simulink model "hexa_CAD_FxQDiff_ASGSM"  (R2024a)
settings: Solver=ode4  StartTime=0.0  StopTime=60  FixedStep=0.01  RelTol=1e-3
undefined symbols (not defined in the file or in its folder): F, Light, MIL, smiData, X, Y, Z
libraries: sm_lib x166, nesl_utility x29, dspobslib x16, sharedtransform x6, aerolibutil x6, simulink x4, sharedutil x2, matrix_library x1, robotcorelib x1, aerolibwind2 x1
(part 2 of 5)

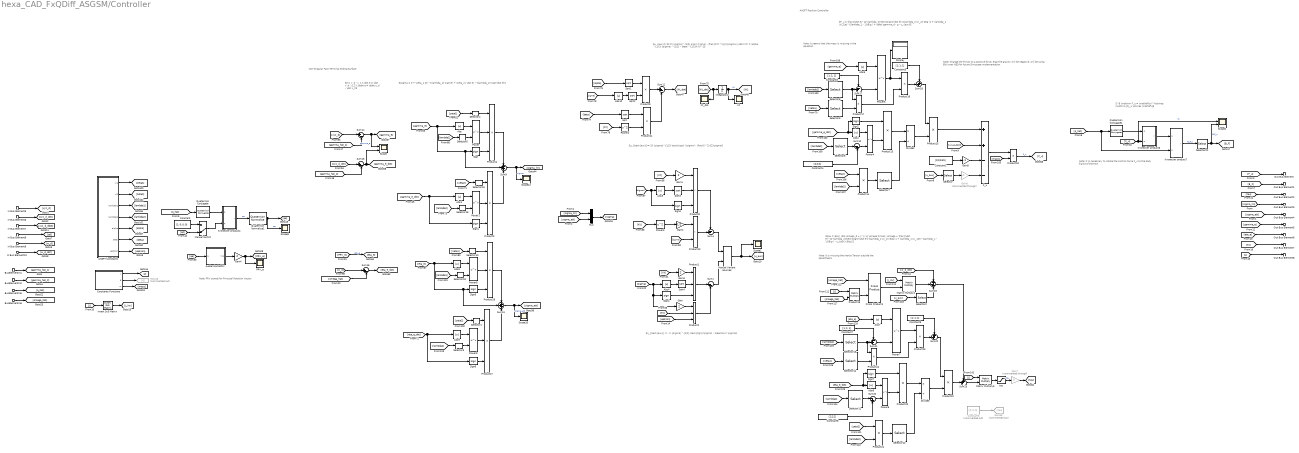
== system hexa_CAD_FxQDiff_ASGSM/Controller ==
  note: $u_{\text{aux}}=-2K |\sigma|^{1/2} \text{sign} (\sigma) - \frac{K^2}{2}\sigma$
  note: $u_{\text{aux}} = - K |\sigma| ^{1/2} \text{sign}(\sigma) - 2\epsilon K \sigma$
  note: Note: PRV stands for Principal Rotation
      | Vector.
  note: $e = x_d - x_1 \\ \dot e = \dot x_d - x_2 \\ \ddot e = \ddot x_d - \dot x_2$
  note: Non-Singular Fast Terminal Sliding Surface
  note: $\sigma = e + \zeta_1 |e| ^{\lambda_1} sign(e) + \zeta_2 | \dot e| ^{\lambda_2} sign(\dot e)$
  note: $F_u = \frac{|\dot e|^{2-\lambda_2}\text{sign}(\dot e)}{\lambda_2 \xi_2} \Big (1 + \lambda_1 \xi_1|e|^{\lambda_1 - 1}\Big ) + \ddot \gamma_d - g - u_{aux}$
  note: Note: It seems that the mass is missing in
      | the equation.
  note: $\tau = \Big [ \dot \omega_d + J^{-1} \omega \times J \omega + \frac{|\dot e|^{2-\lambda_2}\text{sign}(\dot e)}{\lambda_2 \xi_2} \Big (1 + \lambda_1 \xi_1|e|^{\lambda_1 - 1}\Big ) - u_{aux} \Big ]$
  note: Note: Change the Thrust to a positive force, ergo the gravity will be negative,
      | will be using ENU over NED for future Simscape implementation.
  note: $^B \mathrm F_u = \mathbf{q}^*\otimes \mathrm{F}_u \otimes \mathbf q$
  note: ANSFT Position Controller
  note: Note: It is missing the Inertia Tensor outside
      | the parenthesis
  note: Note: It is necessary to rotate the control Force F_u
      | to the body frame of the FAH.
  note: $u_{aux}=-2K(t) |\sigma|^{1/2} sign (\sigma) - \frac{K(t)^2}{2}\sigma \\ \dot K(t) = \alpha ^{1/2} |\sigma| ^{1/2} - \beta ^{1/2}K(t)^2$
  In Bus Element5 : Inport  PortName=chi_d  Element=xyz_d
  In Bus Element6 : Inport  PortName=chi_d  Element=xyz_d_dot
  In Bus Element7 : Inport  PortName=chi_d  Element=xyz_d_ddot
  In Bus Element8 : Inport  PortName=chi_d  Element=qd
  In Bus Element9 : Inport  PortName=chi_d  Element=w_d
  In Bus Element10 : Inport  PortName=chi_d  Element=w_d_dot
  BusElementIn1 : Inport  Port=2  PortName=q_hat  Element=gamma_hat
  BusElementIn2 : Inport  Port=2  PortName=q_hat  Element=gamma_dot_hat
  BusElementIn5 : Inport  Port=2  PortName=q_hat  Element=q_hat
  BusElementIn6 : Inport  Port=2  PortName=q_hat  Element=omega_hat
  ANSFT Constants : MATLAB Function  TreatAsAtomicUnit=on
  Abs{,1..10} (11 alike) : Abs  SaturateOnIntegerOverflow=off
  Constant : Constant  Value=[1; 0; 0; 0]
  Constant1 : Constant  Value=[0;0;9.81]
  Constant{3,5,7,9} (4 alike) : Constant  Value=[1; 1; 1]
  Constant4 : Constant  Value=[2;2;2]
  Constant6 : Constant  Commented=on  Value=[0; 0; 0]
  Constant8 : Constant  Value=[2;2;2]
  Constants Functions : MATLAB Function  TreatAsAtomicUnit=on
  Cross Product1 : matrix_library/Cross Product
  Display : Display
  Divide2 : Product  Inputs=*/
  Divide3 : Product  Inputs=*/
  F_u : Sum  Inputs=++--
  Gain{,1,3..4} (4 alike) : Gain  Gain=2
  Gain2 : Gain  Gain=1/2
  Gain5 : Gain  Gain=-1
  Gain6 : Gain  Commented=through  Gain=-1
  Gain7 : Gain  Commented=through  Gain=0
  Goto18 : Goto  Commented=on  GotoTag=g
  Goto59 : Goto  Commented=on  GotoTag=tau
  Integrator4 : Integrator  InitialCondition=[0;0;0; 0; 0; 0]
  Invert 3x3 Matrix : aerolibutil/Invert  3x3 Matrix
  Kronecker product4 : Subsystem
  Kronecker product6 : Subsystem
  Kronecker product7 : Subsystem
  Kt : Scope
  Kt_dot : Scope
  Manual Variant Source3 : simulink/Signal Routing/Manual Variant Source  NumChoices=2  LabelModeActiveChoice=V_2
  Manual Switch : ManualSwitch  CurrentSetting=0
  Matrix Multiply2 : Product  Multiplication=Matrix(*)
  Matrix Multiply5 : Product  Multiplication=Matrix(*)
  Mux : Mux  Inputs=2
  PRV_e : Scope
  Power{,1,4..9} (8 alike) : Math  Operator=pow
  Power2 : Math  Operator=square
  Power3 : Math  Operator=square
  Product{1..4,8,26..27} (7 alike) : Product  Inputs=3
  Product{9..11,13..18,20..24} (14 alike) : Product
  Product19 : Product  Multiplication=Matrix(*)
  Quaternion Conjugate : aerolibutil/Quaternion Conjugate
  Quaternion Conjugate1 : aerolibutil/Quaternion Conjugate
  Quaternion Normalize1 : sharedutil/Quaternion Normalize  aMode=aMode
  Scope : Scope  NumInputPorts=2
  Scope{1,8,10,12} (4 alike) : Scope
  Scope2 : Scope  NumInputPorts=2
  Selector{,4..9,15..16} (9 alike) : Selector  InputPortWidth=6  IndexOptions=Index vector (dialog)  Indices=[1:3]  OutputSizes=1
  Selector{1..3,10..14,18} (9 alike) : Selector  InputPortWidth=6  IndexOptions=Index vector (dialog)  Indices=[4:6]  OutputSizes=1
  Selector22 : Selector  InputPortWidth=4  IndexOptions=Index vector (dialog)  Indices=[2:4]  OutputSizes=1
  Sign{,1..7} (8 alike) : Signum
  Sqrt{,1..4} (5 alike) : Sqrt
  Sum1 : Sum  Inputs=|--
  Sum10 : Sum  Inputs=|-+
  Sum{11,14..16} (4 alike) : Sum  Inputs=|+-
  Sum17 : Sum  Inputs=-+|
  Sum18 : Sum  Inputs=++|
  Sum19 : Sum  Inputs=+--
  Sum20 : Sum  Inputs=|-+
  Sum21 : Sum  Inputs=-+|
  Sum22 : Sum  Inputs=++|
  Sum23 : Sum  Inputs=++|
  Sum24 : Sum  Inputs=+++
  Sum4 : Sum  Inputs=--|
  Sum9 : Sum  Inputs=+++
  quaterniontoPRV : Subsystem
  tau : Saturate
  Out Bus Element : Outport  PortName=u  Element=F_u
  Out Bus Element1 : Outport  PortName=u  Element=B-F_u
  Out Bus Element2 : Outport  PortName=u  Element=tau
  Out Bus Element3 : Outport  PortName=u  Element=sigma
  Out Bus Element4 : Outport  PortName=u  Element=sigma_att
  Out Bus Element5 : Outport  PortName=u  Element=gamma_e
  Out Bus Element6 : Outport  PortName=u  Element=eta_e
  Out Bus Element7 : Outport  PortName=u  Element=Kt
  Out Bus Element8 : Outport  PortName=u  Element=J
  wires:
  ANSFT Constants/4(lambda2) -> [lambda2]
  ANSFT Constants/6(beta) -> [beta]
  ANSFT Constants/3(lambda1) -> [lambda1]
  ANSFT Constants/1(xi1) -> [zeta1]
  ANSFT Constants/5(alpha) -> [alpha]
  ANSFT Constants/2(xi2) -> [zeta2]
  Constants Functions/1(J) -> [J]
  ANSFT Constants/7(epsilon) -> [epsilon]
  Abs4/1 -> Sqrt4/1
  Gain3/1 -> Product1/1
  Sum4/1 -> Manual Variant Source3/1
  Manual Variant Source3/1 -> Scope1/1, [u_aux]
  Sign4/1 -> Product1/3
  Product8/1 -> Sum4/1
  Product10/1 -> Sum4/2
  Power3/1 -> Gain2/1
  [epsilon] -> Product2/3
  Gain1/1 -> Product8/1
  Gain/1 -> Product2/1
  [Kt] -> Gain1/1
  Product1/1 -> Sum1/1
  Sum1/1 -> Manual Variant Source3/2
  [sigma] -> Product10/2
  Gain2/1 -> Product10/1
  [sigma] -> Abs4/1, Gain/1, Sign4/1
  Sqrt3/1 -> Product8/2
  Product2/1 -> Sum1/2
  Sqrt4/1 -> Product1/2
  [Kt] -> Gain3/1
  [Kt] -> Product2/2
  Abs3/1 -> Sqrt3/1
  [sigma] -> Sign3/1, Abs3/1
  [Kt] -> Power3/1
  Sign3/1 -> Product8/3
  In Bus Element5/1 -> [xyz_d]
  In Bus Element8/1 -> [qd]
  In Bus Element9/1 -> [w_d]
  In Bus Element10/1 -> [w_d_dot]
  In Bus Element6/1 -> [xyz_d_dot]
  In Bus Element7/1 -> [xyz_d_ddot]
  Invert 3x3 Matrix/1 -> [J_inv]
  [J] -> Invert 3x3 Matrix/1
  Kronecker product4/1(r) -> Quaternion Normalize1/1  "qe"
  Constant/1 -> Manual Switch/1
  Gain4/1 -> PRV_e/1, [PRV_e]
  [q_hat] -> Quaternion Conjugate/1
  Quaternion Conjugate/1 -> Kronecker product4/1(q)
  [qe] -> quaterniontoPRV/1(q)
  Quaternion Normalize1/1 -> Scope8/1, [qe]  "qe"
  [qd] -> Manual Switch/2
  quaterniontoPRV/1(lnq) -> Gain4/1
  Manual Switch/1 -> Kronecker product4/2(p)
  [eta_e] -> Sum24/2, Sign5/1, Abs8/1
  Selector18/1 -> Power8/2
  Sum24/1 -> Scope10/1, [sigma_att]  "sigma_att"
  Sum15/1 -> Scope/2, [gamma_e_dot]
  [xyz_d] -> Sum14/1
  Sign/1 -> Product4/3
  Selector4/1 -> Product4/1
  Power/1 -> Product4/2
  Selector3/1 -> Power9/2
  [xyz_d_dot] -> Sum15/1
  Product27/1 -> Sum24/3
  [PRV_e] -> [eta_e]  "eta_e"
  [zeta2] -> Selector1/1
  [lambda2] -> Selector16/1
  Abs8/1 -> Power8/1
  [eta_e_dot] -> Abs9/1, Sign6/1
  Selector16/1 -> Power1/2
  Product26/1 -> Sum24/1
  [lambda2] -> Selector3/1
  [gamma_e_dot] -> Sign1/1, Abs1/1
  [gamma_hat_1] -> Sum14/2
  Sign5/1 -> Product26/3
  [gamma_e] -> Sum9/2, Sign/1, Abs/1
  Sign1/1 -> Product3/3
  [gamma_hat_2] -> Sum15/2
  Sum9/1 -> Scope12/1, [sigma_lin]  "sigma"
  [omega_hat] -> Sum16/2
  [zeta2] -> Selector15/1
  [lambda1] -> Selector5/1
  [w_d] -> Sum16/1
  Selector5/1 -> Power/2
  Power9/1 -> Product27/2
  [zeta1] -> Selector10/1
  Abs9/1 -> Power9/1
  [zeta1] -> Selector4/1
  Abs/1 -> Power/1
  Sum14/1 -> Scope/1, [gamma_e]  "gamma_e"
  [lambda1] -> Selector18/1
  Power1/1 -> Product3/2
  Selector10/1 -> Product26/1
  Product4/1 -> Sum9/1
  Selector1/1 -> Product27/1
  Sum16/1 -> [eta_e_dot]
  Sign6/1 -> Product27/3
  Product3/1 -> Sum9/3
  Abs1/1 -> Power1/1
  Selector15/1 -> Product3/1
  Power8/1 -> Product26/2
  [sigma_lin] -> Mux/1
  [sigma_att] -> Mux/2
  Mux/1 -> [sigma]
  Sum20/1 -> Power6/2
  Product13/1 -> Divide2/1
  Product20/1 -> Divide3/1
  Sum21/1 -> Power7/2
  Constant9/1 -> Sum22/1
  Selector8/1 -> Product17/1, Sum17/2
  [w_d_dot] -> Sum19/1
  Abs2/1 -> Power4/1
  [eta_e_dot] -> Sign7/1, Abs6/1
  [zeta2] -> Product14/1
  Constant3/1 -> Sum17/1
  [eta_e] -> Abs7/1
  Abs7/1 -> Power7/1
  Selector7/1 -> Divide2/2
  [zeta1] -> Selector14/1
  Constant8/1 -> Sum20/2
  Product23/1 -> Sum22/2
  Matrix Multiply5/1 -> tau/1
  Selector14/1 -> Product24/2
  Selector9/1 -> Product17/2
  Sum10/1 -> Power4/2
  Abs5/1 -> Power5/1
  [zeta2] -> Product21/1
  Kronecker product6/1(r) -> Kronecker product7/1(q)
  [lambda2] -> Product14/2
  [lambda1] -> Selector8/1
  Constant1/1 -> Gain5/1
  [J] -> Matrix Multiply5/1
  Sum18/1 -> Product15/1
  [zeta1] -> Selector9/1
  Selector12/1 -> Divide3/2
  Selector13/1 -> Product24/1, Sum21/2
  Power5/1 -> Display/1, Product16/1
  Product15/1 -> F_u/1
  Constant7/1 -> Sum21/1
  Selector6/1 -> Sum10/1
  [u_aux] -> Selector/1
  Product24/1 -> Product23/2
  Sign7/1 -> Product20/1
  [xyz_d_ddot] -> F_u/2
  Sign2/1 -> Product13/1
  Product21/1 -> Selector12/1
  [lambda2] -> Selector6/1
  [lambda2] -> Product21/2
  F_u/1 -> Product18/1
  Product22/1 -> Sum23/2
  [mass] -> Product18/2
  Product14/1 -> Selector7/1
  Abs6/1 -> Power6/1
  Product16/1 -> Sum18/2
  [gamma_e_dot] -> Sign2/1, Abs2/1
  Product18/1 -> [F_u]  "F_u"
  Selector22/1 -> Scope2/2, [B_F]  "B-F_u"
  Constant4/1 -> Sum10/2
  Power4/1 -> Product13/2
  [lambda2] -> Selector11/1
  Divide3/1 -> Product22/2
  Gain6/1 -> F_u/4
  Selector11/1 -> Sum20/1
  Divide2/1 -> Product15/2
  Sum19/1 -> Sum23/1
  [gamma_e] -> Abs5/1
  Product17/1 -> Product16/2
  Sum22/1 -> Product22/1
  Sum23/1 -> Matrix Multiply5/2
  Constant5/1 -> Sum18/1
  [F_u] -> Scope2/1, Kronecker product6/2(p)  "fu"
  [lambda1] -> Selector13/1
  Constant6/1 -> Goto59/1
  [u_aux] -> Selector2/1
  tau/1 -> Gain7/1  "tau"
  [q_hat] -> Kronecker product7/2(p), Quaternion Conjugate1/1
  Quaternion Conjugate1/1 -> Kronecker product6/1(q)
  Kronecker product7/1(r) -> Selector22/1  "B_F_u"
  Sum17/1 -> Power5/2
  Power6/1 -> Product20/2
  Power7/1 -> Product23/1
  [B_F] -> Out Bus Element1/1
  [Kt] -> Out Bus Element7/1
  [eta_e] -> Out Bus Element6/1
  [sigma_lin] -> Out Bus Element3/1
  [gamma_e] -> Out Bus Element5/1
  [tau] -> Out Bus Element2/1
  [sigma_att] -> Out Bus Element4/1
  [F_u] -> Out Bus Element/1
  Integrator4/1 -> Kt/1, [Kt]  "Kt"
  Product9/1 -> Sum11/1
  [Kt_dot] -> Kt_dot/1, Integrator4/1
  [beta] -> Sqrt/1
  [sigma] -> Abs10/1
  [alpha] -> Sqrt1/1
  Sqrt1/1 -> Product9/1
  Product11/1 -> Sum11/2
  Abs10/1 -> Sqrt2/1
  Sqrt2/1 -> Product9/2
  [Kt] -> Power2/1
  Sum11/1 -> [Kt_dot]
  Sqrt/1 -> Product11/1
  Power2/1 -> Product11/2
  Constants Functions/2(g) -> Goto18/1
  Constants Functions/3(m) -> [mass]
  Selector/1 -> Gain6/1
  Selector2/1 -> Sum19/3
  [J] -> Out Bus Element8/1
  BusElementIn1/1 -> [gamma_hat_1]
  BusElementIn2/1 -> [gamma_hat_2]
  BusElementIn6/1 -> [omega_hat]
  BusElementIn5/1 -> [q_hat]
  [J] -> Product19/1
  [omega_hat] -> Cross Product1/1
  Cross Product1/1 -> Matrix Multiply2/2
  [J_inv] -> Matrix Multiply2/1
  Matrix Multiply2/1 -> Sum19/2
  [omega_hat] -> Product19/2
  Product19/1 -> Cross Product1/2
  Gain5/1 -> F_u/3
  Gain7/1 -> [tau]

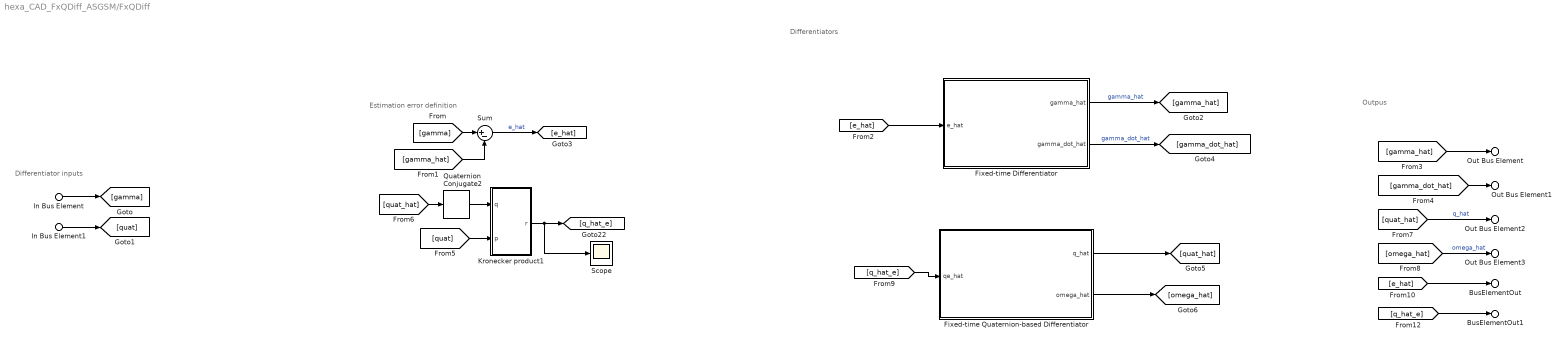
== system hexa_CAD_FxQDiff_ASGSM/FxQDiff ==
  note: Outpus
  note: Differentiators
  note: Differentiator inputs
  note: Estimation error definition
  In Bus Element : Inport  PortName=chi  Element=pos
  In Bus Element1 : Inport  PortName=chi  Element=q
  Fixed-time Differentiator : Subsystem
  Fixed-time Quaternion-based Differentiator : Subsystem
  Kronecker product1 : Subsystem
  Quaternion Conjugate2 : aerolibutil/Quaternion Conjugate
  Scope : Scope
  Sum : Sum  Inputs=|+-
  Out Bus Element : Outport  PortName=chi_hat  Element=gamma_hat
  Out Bus Element1 : Outport  PortName=chi_hat  Element=gamma_dot_hat
  Out Bus Element2 : Outport  PortName=chi_hat  Element=q_hat
  Out Bus Element3 : Outport  PortName=chi_hat  Element=omega_hat
  BusElementOut : Outport  PortName=chi_hat  Element=e_hat
  BusElementOut1 : Outport  PortName=chi_hat  Element=qe_hat
  wires:
  [gamma] -> Sum/1
  [gamma_hat] -> Sum/2
  Sum/1 -> [e_hat]  "e_hat"
  [e_hat] -> Fixed-time Differentiator/1(e_hat)
  Fixed-time Differentiator/1(gamma_hat) -> [gamma_hat]  "gamma_hat"
  Fixed-time Differentiator/2(gamma_dot_hat) -> [gamma_dot_hat]  "gamma_dot_hat"
  In Bus Element/1 -> [gamma]
  In Bus Element1/1 -> [quat]
  [gamma_hat] -> Out Bus Element/1
  [gamma_dot_hat] -> Out Bus Element1/1
  Quaternion Conjugate2/1 -> Kronecker product1/1(q)
  [quat_hat] -> Out Bus Element2/1  "q_hat"
  [omega_hat] -> Out Bus Element3/1  "omega_hat"
  [q_hat_e] -> Fixed-time Quaternion-based Differentiator/1(qe_hat)
  Fixed-time Quaternion-based Differentiator/1(q_hat) -> [quat_hat]
  Fixed-time Quaternion-based Differentiator/2(omega_hat) -> [omega_hat]
  Kronecker product1/1(r) -> Scope/1, [q_hat_e]
  [e_hat] -> BusElementOut/1
  [q_hat_e] -> BusElementOut1/1
  [quat_hat] -> Quaternion Conjugate2/1
  [quat] -> Kronecker product1/2(p)

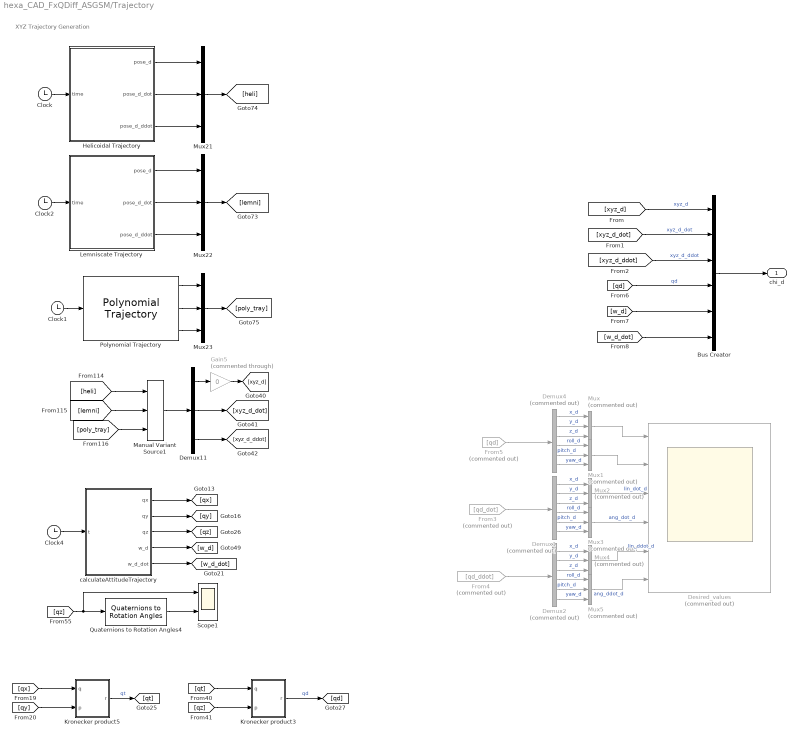
== system hexa_CAD_FxQDiff_ASGSM/Trajectory ==
  note: XYZ Trajectory Generation
  Bus Creator : BusCreator  Inputs=6
  Clock{,1..2,4} (4 alike) : Clock
  Demux1 : Demux  Commented=on  Outputs=6
  Demux11 : Demux  Outputs=3
  Demux2 : Demux  Commented=on  Outputs=6
  Demux4 : Demux  Commented=on  Outputs=6
  Desired_values : Scope  Commented=on  NumInputPorts=6
  From3 : From  Commented=on  GotoTag=qd_dot
  From4 : From  Commented=on  GotoTag=qd_ddot
  From5 : From  Commented=on  GotoTag=qd
  Gain5 : Gain  Commented=through  Gain=0
  Helicoidal Trajectory : MATLAB Function  TreatAsAtomicUnit=on
  Kronecker product3 : Subsystem
  Kronecker product5 : Subsystem
  Lemniscate Trajectory : MATLAB Function  TreatAsAtomicUnit=on
  Manual Variant Source1 : simulink/Signal Routing/Manual Variant Source  NumChoices=3  LabelModeActiveChoice=V_1
  Mux{,1..5} (6 alike) : Mux  Commented=on  Inputs=3
  Mux21 : Mux  Inputs=3
  Mux22 : Mux  Inputs=3
  Mux23 : Mux  Inputs=3
  Polynomial Trajectory : robotcorelib/Polynomial Trajectory  WaypointSource=Internal  Waypoints=zeros(3, 6)  TimePoints=[ 0, 12, 24, 36, 48, 60]  TimeInterval=[ 1, 4 ]  Method=Cubic Polynomial  ParameterSource=Internal  VelocityBoundaryCondition=zeros( 3, 6)  AccelerationBoundaryCondition=zeros( 2, 5 )  SimulateUsing=Interpreted execution
  Quaternions to Rotation Angles4 : sharedtransform/Quaternions to Rotation Angles  rotationOrder=ZYX  aMode=aMode
  Scope1 : Scope  NumInputPorts=2
  calculateAttitudeTrajectory : MATLAB Function  TreatAsAtomicUnit=on
  chi_d : Outport
  wires:
  Demux4/1 -> Mux/1  "x_d"
  Demux2/5 -> Mux5/2  "pitch_d"
  Demux1/5 -> Mux3/2  "pitch_d"
  Demux1/3 -> Mux2/3  "z_d"
  Demux4/6 -> Mux1/3  "yaw_d"
  From3/1 -> Demux1/1
  Demux1/2 -> Mux2/2  "y_d"
  Mux1/1 -> Desired_values/2
  Demux4/3 -> Mux/3  "z_d"
  Demux4/2 -> Mux/2  "y_d"
  Demux1/1 -> Mux2/1  "x_d"
  From4/1 -> Demux2/1
  Mux2/1 -> Desired_values/3  "lin_dot_d"
  Demux4/5 -> Mux1/2  "pitch_d"
  Mux5/1 -> Desired_values/6  "ang_ddot_d"
  Demux2/3 -> Mux4/3  "z_d"
  From5/1 -> Demux4/1
  Mux3/1 -> Desired_values/4  "ang_dot_d"
  Demux4/4 -> Mux1/1  "roll_d"
  Mux/1 -> Desired_values/1
  Demux1/4 -> Mux3/1  "roll_d"
  Demux2/1 -> Mux4/1  "x_d"
  Demux1/6 -> Mux3/3  "yaw_d"
  Mux4/1 -> Desired_values/5  "lin_ddot_d"
  Bus Creator/1 -> chi_d/1
  Demux2/4 -> Mux5/1  "roll_d"
  Demux2/6 -> Mux5/3  "yaw_d"
  Demux2/2 -> Mux4/2  "y_d"
  [lemni] -> Manual Variant Source1/2
  Clock1/1 -> Polynomial Trajectory/1
  Gain5/1 -> [xyz_d]
  calculateAttitudeTrajectory/3(qz) -> [qz]
  Helicoidal Trajectory/1(pose_d) -> Mux21/1
  [poly_tray] -> Manual Variant Source1/3
  [qz] -> Scope1/1, Quaternions to Rotation Angles4/1
  Polynomial Trajectory/3 -> Mux23/3
  Helicoidal Trajectory/2(pose_d_dot) -> Mux21/2
  Demux11/1 -> Gain5/1
  Demux11/3 -> [xyz_d_ddot]
  Clock4/1 -> calculateAttitudeTrajectory/1(t)
  Lemniscate Trajectory/2(pose_d_dot) -> Mux22/2
  calculateAttitudeTrajectory/1(qx) -> [qx]
  calculateAttitudeTrajectory/2(qy) -> [qy]
  calculateAttitudeTrajectory/5(w_d_dot) -> [w_d_dot]
  Clock/1 -> Helicoidal Trajectory/1(time)
  [heli] -> Manual Variant Source1/1
  calculateAttitudeTrajectory/4(w_d) -> [w_d]
  Polynomial Trajectory/1 -> Mux23/1
  Clock2/1 -> Lemniscate Trajectory/1(time)
  Demux11/2 -> [xyz_d_dot]
  Mux22/1 -> [lemni]
  Helicoidal Trajectory/3(pose_d_ddot) -> Mux21/3
  Lemniscate Trajectory/3(pose_d_ddot) -> Mux22/3
  Lemniscate Trajectory/1(pose_d) -> Mux22/1
  Mux23/1 -> [poly_tray]
  Manual Variant Source1/1 -> Demux11/1
  Quaternions to Rotation Angles4/1 -> Scope1/2
  Polynomial Trajectory/2 -> Mux23/2
  Mux21/1 -> [heli]
  [w_d_dot] -> Bus Creator/6
  [qd] -> Bus Creator/4  "qd"
  [w_d] -> Bus Creator/5
  [xyz_d_ddot] -> Bus Creator/3  "xyz_d_ddot"
  [xyz_d_dot] -> Bus Creator/2  "xyz_d_dot"
  [xyz_d] -> Bus Creator/1  "xyz_d"
  [qx] -> Kronecker product5/1(q)
  Kronecker product3/1(r) -> [qd]  "qd"
  [qz] -> Kronecker product3/2(p)
  [qt] -> Kronecker product3/1(q)
  Kronecker product5/1(r) -> [qt]  "qt"
  [qy] -> Kronecker product5/2(p)

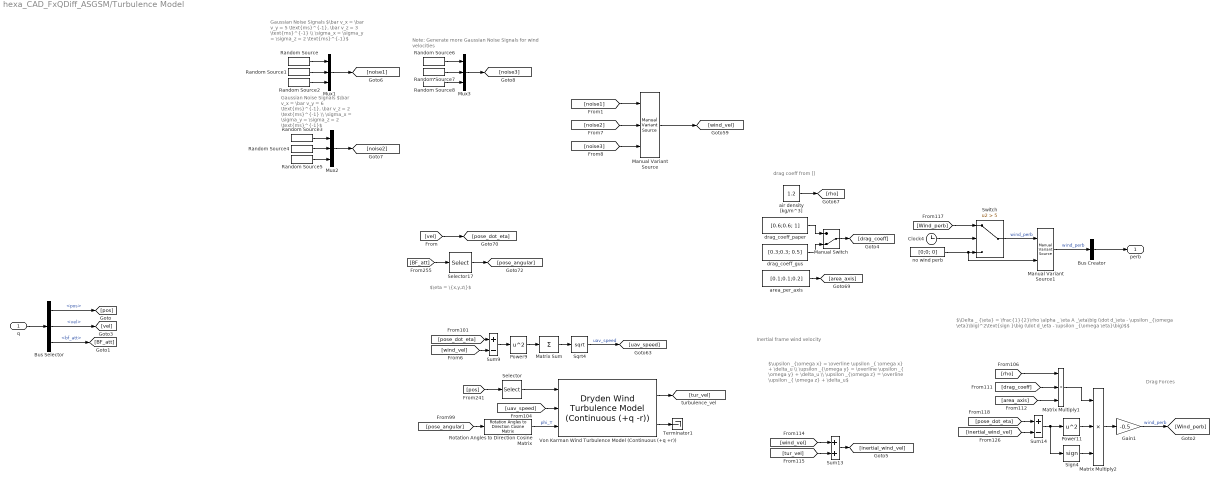
== system hexa_CAD_FxQDiff_ASGSM/Turbulence Model ==
  note: Note: Generate more Gaussian Noise Signals
      | for wind velocities
  note: $\Delta _ {\eta} = \frac{1}{2}\rho \alpha _ \eta A _\eta\big (\dot d_\eta - \upsilon _{\omega \eta}\big)^2\text{sign }\big (\dot d_\eta - \upsilon _{\omega \eta}\big)$$
  note: $\upsilon _{\omega x} = \overline \upsilon _{ \omega x} + \delta_u \\ \upsilon _{\omega y} = \overline \upsilon _{ \omega y} + \delta_u \\ \upsilon _{\omega z} = \overline \upsilon _{ \omega z} + \delta_u$
  note: drag coeff from []
  note: Drag Forces
  note: Inertial frame wind velocity
  note: $\eta = \{x,y,z\}$
  note: Gaussian Noise Signals
      | $\bar v_x = \bar v_y = 6 \text{ms}^{-1}, \bar v_z = 2 \text{ms}^{-1} \\ \sigma_x = \sigma_y = \sigma_z = 2 \text{ms}^{-1}$
  note: Gaussian Noise Signals
      | $\bar v_x = \bar v_y = 5 \text{ms}^{-1}, \bar v_z = 3 \text{ms}^{-1} \\ \sigma_x = \sigma_y = \sigma_z = 2 \text{ms}^{-1}$
  q : Inport
  Bus Creator : BusCreator  Inputs=1
  Bus Selector : BusSelector  OutputSignals=pos,vel,bf_att
  Clock4 : Clock
  Gain1 : Gain  Gain=-0.5
  Manual Variant Source : simulink/Signal Routing/Manual Variant Source  NumChoices=3  LabelModeActiveChoice=V_1
  Manual Variant Source1 : simulink/Signal Routing/Manual Variant Source  NumChoices=2  LabelModeActiveChoice=V_1
  Manual Switch : ManualSwitch  CurrentSetting=0
  Matrix Sum : Sum  Inputs=+
  Matrix Multiply1 : Product  Inputs=3
  Matrix Multiply2 : Product  Inputs=3
  Mux1 : Mux  Inputs=3
  Mux2 : Mux  Inputs=3
  Mux3 : Mux  Inputs=3
  Power11 : Math  Operator=square
  Power9 : Math  Operator=square
  Random Source : dspobslib/Random Source  SrcType=Gaussian  NormMethod=Ziggurat  CltLength=12  MinVal=0  MaxVal=1  MeanVal=5  VarVal=2  RepMode=Not repeatable  rawSeed=1  IsInherit=off  SampMode=Discrete  SampTime=1  SampFrame=1  DataType=Double  OutComplex=Real  OutputFrames=off
  Random Source1 : dspobslib/Random Source  SrcType=Gaussian  NormMethod=Ziggurat  CltLength=12  MinVal=0  MaxVal=1  MeanVal=5  VarVal=2  RepMode=Not repeatable  rawSeed=1  IsInherit=off  SampMode=Discrete  SampTime=1  SampFrame=1  DataType=Double  OutComplex=Real  OutputFrames=off
  Random Source2 : dspobslib/Random Source  SrcType=Gaussian  NormMethod=Ziggurat  CltLength=12  MinVal=0  MaxVal=1  MeanVal=3  VarVal=2  RepMode=Not repeatable  rawSeed=1  IsInherit=off  SampMode=Discrete  SampTime=1  SampFrame=1  DataType=Double  OutComplex=Real  OutputFrames=off
  Random Source{3..4,6..7} (4 alike) : dspobslib/Random Source  SrcType=Gaussian  NormMethod=Ziggurat  CltLength=12  MinVal=0  MaxVal=1  MeanVal=6  VarVal=2  RepMode=Not repeatable  rawSeed=1  IsInherit=off  SampMode=Discrete  SampTime=1  SampFrame=1  DataType=Double  OutComplex=Real  OutputFrames=off
  Random Source5 : dspobslib/Random Source  SrcType=Gaussian  NormMethod=Ziggurat  CltLength=12  MinVal=0  MaxVal=1  MeanVal=2  VarVal=2  RepMode=Not repeatable  rawSeed=1  IsInherit=off  SampMode=Discrete  SampTime=1  SampFrame=1  DataType=Double  OutComplex=Real  OutputFrames=off
  Random Source8 : dspobslib/Random Source  SrcType=Gaussian  NormMethod=Ziggurat  CltLength=12  MinVal=0  MaxVal=1  MeanVal=2  VarVal=2  RepMode=Not repeatable  rawSeed=1  IsInherit=off  SampMode=Discrete  SampTime=1  SampFrame=1  DataType=Double  OutComplex=Real  OutputFrames=off
  Rotation Angles to Direction Cosine Matrix : sharedtransform/Rotation Angles to Direction Cosine Matrix  rotationOrder=XYZ  aMode=aMode
  Selector : Selector  InputPortWidth=3  IndexOptions=Index vector (dialog)  Indices=[3]  OutputSizes=1
  Selector17 : Selector  InputPortWidth=3  IndexOptions=Index vector (dialog)  Indices=[3 2 1]  OutputSizes=1
  Sign4 : Signum
  Sqrt4 : Sqrt
  Sum13 : Sum
  Sum14 : Sum  Inputs=+-
  Sum9 : Sum  Inputs=+-
  Switch : Switch  Criteria=u2 > Threshold  Threshold=5  SaturateOnIntegerOverflow=off  InputSameDT=off
  Terminator1 : Terminator
  Von Karman Wind Turbulence Model (Continuous (+q +r)) : aerolibwind2/Dryden Wind Turbulence Model  (Continuous (+q -r))  units=Metric (MKS)  spec=MIL-F-8785C  model=Continuous Von Karman (+q -r)  W20=15  Wdeg=0  TurbProb=10^-2 - Light  L_high=762  Wingspan=10  ts=0.1  Seed=[23341 23342 23343 23344]  T_on=on
      settings: LibrarySourceBlock=|
      | aerolibwind2/Von Karman Wind Turbulence Model
      | (Continuous (+q +r))
  air density [kg/m^3] : Constant  Value=1.2
  area_per_axis : Constant  Value=[0.1;0.1;0.2]
  drag_coeff_gus : Constant  Value=[0.3;0.3; 0.5]
  drag_coeff_paper : Constant  Value=[0.6;0.6; 1]
  no wind perb : Constant  Value=[0;0; 0]
  perb : Outport
  wires:
  [rho] -> Matrix Multiply1/1
  [drag_coeff] -> Matrix Multiply1/2
  Von Karman Wind Turbulence Model (Continuous (+q +r))/2 -> Terminator1/1
  area_per_axis/1 -> [area_axis]
  [pose_dot_eta] -> Sum14/1
  Von Karman Wind Turbulence Model (Continuous (+q +r))/1 -> [tur_vel]
  [wind_vel] -> Sum9/2
  Selector17/1 -> [pose_angular]
  Matrix Multiply1/1 -> Matrix Multiply2/1
  Sign4/1 -> Matrix Multiply2/3
  [uav_speed] -> Von Karman Wind Turbulence Model (Continuous (+q +r))/2
  Power9/1 -> Matrix Sum/1
  Sqrt4/1 -> [uav_speed]  "uav_speed"
  Gain1/1 -> [Wind_perb]  "wind_perb"
  Sum9/1 -> Power9/1
  air density [kg/m^3]/1 -> [rho]
  Clock4/1 -> Switch/2
  [pose_dot_eta] -> Sum9/1
  Rotation Angles to Direction Cosine Matrix/1 -> Von Karman Wind Turbulence Model (Continuous (+q +r))/3  "phi_T"
  [tur_vel] -> Sum13/2
  Sum14/1 -> Sign4/1, Power11/1
  no wind perb/1 -> Manual Variant Source1/2, Switch/3
  drag_coeff_gus/1 -> Manual Switch/2
  Switch/1 -> Manual Variant Source1/1  "wind_perb"
  [area_axis] -> Matrix Multiply1/3
  Manual Switch/1 -> [drag_coeff]
  Selector/1 -> Von Karman Wind Turbulence Model (Continuous (+q +r))/1
  [pose_angular] -> Rotation Angles to Direction Cosine Matrix/1
  [inertial_wind_vel] -> Sum14/2
  Matrix Multiply2/1 -> Gain1/1
  drag_coeff_paper/1 -> Manual Switch/1
  Power11/1 -> Matrix Multiply2/2
  Matrix Sum/1 -> Sqrt4/1
  Sum13/1 -> [inertial_wind_vel]
  [Wind_perb] -> Switch/1
  [wind_vel] -> Sum13/1
  Bus Creator/1 -> perb/1
  [BF_att] -> Selector17/1
  [pos] -> Selector/1
  q/1 -> Bus Selector/1
  Bus Selector/1 -> [pos]  "<pos>"
  Bus Selector/3 -> [BF_att]  "<bf_att>"
  Bus Selector/2 -> [vel]  "<vel>"
  [vel] -> [pose_dot_eta]
  Mux2/1 -> [noise2]
  Random Source5/1 -> Mux2/3
  Random Source/1 -> Mux1/1
  Mux1/1 -> [noise1]
  Random Source2/1 -> Mux1/3
  Random Source4/1 -> Mux2/2
  Random Source3/1 -> Mux2/1
  [noise2] -> Manual Variant Source/2
  Manual Variant Source/1 -> [wind_vel]
  Random Source1/1 -> Mux1/2
  [noise1] -> Manual Variant Source/1
  [noise3] -> Manual Variant Source/3
  Mux3/1 -> [noise3]
  Random Source7/1 -> Mux3/2
  Random Source6/1 -> Mux3/1
  Random Source8/1 -> Mux3/3
  Manual Variant Source1/1 -> Bus Creator/1  "wind_perb"

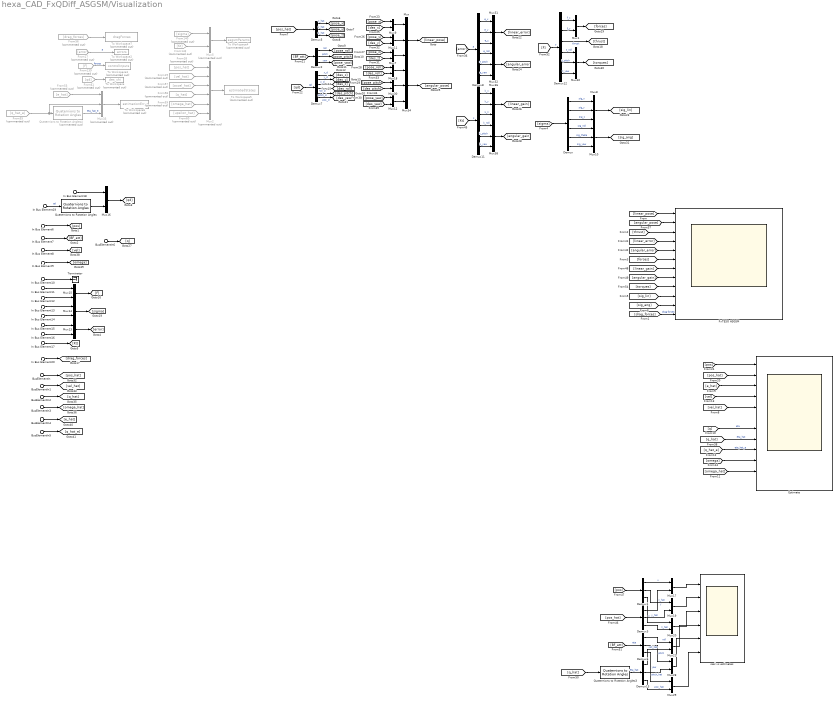
== system hexa_CAD_FxQDiff_ASGSM/Visualization ==
  In Bus Element6 : Inport  PortName=q  Element=pos
  In Bus Element7 : Inport  PortName=q  Element=bf_att
  In Bus Element8 : Inport  PortName=q  Element=vel
  In Bus Element9 : Inport  PortName=q  Element=bf_datt
  BusElementIn6 : Inport  PortName=q  Element=q
  In Bus Element18 : Inport  Port=2  PortName=qd  Element=xyz_d
  In Bus Element19 : Inport  Port=2  PortName=qd  Element=qd
  In Bus Element10 : Inport  Port=3  PortName=u  Element=F_u
  In Bus Element11 : Inport  Port=3  PortName=u  Element=B-F_u
  In Bus Element12 : Inport  Port=3  PortName=u  Element=tau
  In Bus Element13 : Inport  Port=3  PortName=u  Element=sigma
  In Bus Element14 : Inport  Port=3  PortName=u  Element=sigma_att
  In Bus Element15 : Inport  Port=3  PortName=u  Element=gamma_e
  In Bus Element16 : Inport  Port=3  PortName=u  Element=eta_e
  In Bus Element17 : Inport  Port=3  PortName=u  Element=Kt
  In Bus Element20 : Inport  Port=4  PortName=perb  Element=wind_perb
  BusElementIn : Inport  Port=5  PortName=q_hat  Element=gamma_hat
  BusElementIn1 : Inport  Port=5  PortName=q_hat  Element=gamma_dot_hat
  BusElementIn2 : Inport  Port=5  PortName=q_hat  Element=q_hat
  BusElementIn3 : Inport  Port=5  PortName=q_hat  Element=omega_hat
  BusElementIn4 : Inport  Port=5  PortName=q_hat  Element=e_hat
  BusElementIn5 : Inport  Port=5  PortName=q_hat  Element=qe_hat
  Demux{,7..8,11..12} (5 alike) : Demux  Outputs=6
  Demux{1..3,5..6,13} (6 alike) : Demux  Outputs=3
  Estimate : Scope  NumInputPorts=12
  From139 : From  Commented=on  GotoTag=F
  From140 : From  Commented=on  GotoTag=sigma
  From142 : From  Commented=on  GotoTag=Kt
  From17 : From  Commented=on  GotoTag=error
  From18 : From  Commented=on  GotoTag=pos_hat
  From19 : From  Commented=on  GotoTag=vel_hat
  From53 : From  Commented=on  GotoTag=e_hat
  From55 : From  Commented=on  GotoTag=q_hat_e
  From56 : From  Commented=on  GotoTag=drag_forces
  From57 : From  Commented=on  GotoTag=accel_hat
  From58 : From  Commented=on  GotoTag=q_hat
  From59 : From  Commented=on  GotoTag=omega_hat
  From60 : From  Commented=on  GotoTag=upsilon_hat
  From61 : From  Commented=on  GotoTag=qd
  FxTESO ASGSM : Scope  NumInputPorts=12
  Mux{,8,10,31..32,34,36,38,40} (9 alike) : Mux  Inputs=3
  Mux{1,7,9,11..21,28..30} (17 alike) : Mux  Inputs=2
  Mux2 : Mux  Commented=on  Inputs=6
  Mux33 : Mux  Commented=on  Inputs=3
  Mux5 : Mux  Commented=on  Inputs=2
  Quaternions to Rotation Angles : sharedtransform/Quaternions to Rotation Angles  rotationOrder=XYZ  aMode=aMode
  Quaternions to Rotation Angles3 : sharedtransform/Quaternions to Rotation Angles  rotationOrder=XYZ  aMode=aMode
  Quaternions to Rotation Angles4 : sharedtransform/Quaternions to Rotation Angles  Commented=on  rotationOrder=XYZ  aMode=aMode
  Terminator : Terminator
  To Workspace : ToWorkspace  Commented=on  VariableName=des_chi  SaveFormat=Structure With Time  SampleTime=-1
  To Workspace2 : ToWorkspace  Commented=on  VariableName=errors  SaveFormat=Structure With Time  SampleTime=-1
  To Workspace3 : ToWorkspace  Commented=on  VariableName=controlInputs  SaveFormat=Structure With Time  SampleTime=-1
  To Workspace4 : ToWorkspace  Commented=on  VariableName=asgsmParams  SaveFormat=Structure With Time  SampleTime=-1
  To Workspace5 : ToWorkspace  Commented=on  VariableName=estimatedStates  SaveFormat=Timeseries  SampleTime=-1
  To Workspace6 : ToWorkspace  Commented=on  VariableName=estimationError  SaveFormat=Structure With Time  SampleTime=-1
  To Workspace7 : ToWorkspace  Commented=on  VariableName=dragForces  SaveFormat=Timeseries  SampleTime=-1
  real vs estimates : Scope  NumInputPorts=6
  wires:
  Mux/1 -> [linear_pose]
  Mux9/1 -> Mux/1
  Demux7/5 -> [des_pitch]  "pitch_d"
  [linear_error] -> FxTESO ASGSM/4
  [angular_error] -> FxTESO ASGSM/5
  Mux11/1 -> Mux/2
  Demux11/2 -> Mux36/2  "k_y"
  Demux5/1 -> [pose_x]  "x_hat"
  Demux12/6 -> Mux40/3  "t_yaw"
  Demux12/4 -> Mux40/1  "t_roll"
  Mux40/1 -> [torques]
  Mux1/1 -> [forces]
  Demux5/3 -> [pose_z]  "z_hat"
  Demux11/1 -> Mux36/1  "k_x"
  Demux8/6 -> Mux32/3  "e_yaw"
  Demux11/4 -> Mux38/1  "k_roll"
  [BF_att] -> Demux2/1
  Mux31/1 -> [linear_error]
  Demux7/2 -> [des_y]  "y_d"
  Demux5/2 -> [pose_y]  "y_hat"
  [pose_pitch] -> Mux30/1
  [pose_y] -> Mux11/1
  Demux8/3 -> Mux31/3  "e_z"
  Demux7/3 -> [des_z]  "z_d"
  Demux12/2 -> Mux1/2  "f_y"
  [angular_gain] -> FxTESO ASGSM/8
  [error] -> Demux8/1  "e"
  [des_pitch] -> Mux30/2
  [F] -> Demux12/1  "f"
  Mux5/1 -> To Workspace4/1
  [linear_gain] -> FxTESO ASGSM/7
  From61/1 -> To Workspace/1
  [des_roll] -> Mux18/2
  Demux12/1 -> Mux1/1  "f_x"
  Demux7/4 -> [des_roll]  "roll_d"
  Demux12/3 -> [thrust]  "thrust"
  Mux36/1 -> [linear_gain]
  [des_yaw] -> Mux12/2
  Demux11/6 -> Mux38/3  "k_yaw"
  From139/1 -> To Workspace3/1  "forces"
  [angular_pose] -> FxTESO ASGSM/2
  Demux8/1 -> Mux31/1  "e_x"
  Demux7/1 -> [des_x]  "x_d"
  [pose_yaw] -> Mux12/1
  Mux12/1 -> Mux34/3
  Demux12/5 -> Mux40/2  "t_pitch"
  [des_x] -> Mux9/2
  Demux8/4 -> Mux32/1  "e_roll"
  [linear_pose] -> FxTESO ASGSM/1
  Mux7/1 -> Mux/3
  From17/1 -> To Workspace2/1  "e"
  Demux8/5 -> Mux32/2  "e_pitch"
  Mux34/1 -> [angular_pose]
  [pose_x] -> Mux9/1
  [pose_roll] -> Mux18/1
  [pose_z] -> Mux7/1
  Mux30/1 -> Mux34/2
  [des_y] -> Mux11/2
  Demux11/3 -> Mux36/3  "k_z"
  Demux7/6 -> [des_yaw]  "yaw_d"
  Mux38/1 -> [angular_gain]
  Mux18/1 -> Mux34/1
  Demux11/5 -> Mux38/2  "k_pitch"
  [Kt] -> Demux11/1  "k"
  Mux32/1 -> [angular_error]
  [qd] -> Demux7/1  "qd"
  Demux8/2 -> Mux31/2  "e_y"
  [des_z] -> Mux7/2
  From142/1 -> Mux5/2
  From140/1 -> Mux5/1
  In Bus Element6/1 -> [pos]
  In Bus Element7/1 -> [BF_att]
  In Bus Element10/1 -> Terminator/1
  In Bus Element11/1 -> Mux15/1
  In Bus Element12/1 -> Mux15/2
  In Bus Element20/1 -> [drag_forces]
  [thrust] -> FxTESO ASGSM/3
  [forces] -> FxTESO ASGSM/6
  [torques] -> FxTESO ASGSM/9
  [drag_forces] -> FxTESO ASGSM/12  "drag forces"
  In Bus Element13/1 -> Mux14/1
  Demux/6 -> Mux10/3  "sig_yaw"
  Demux/5 -> Mux10/2  "sig_theta"
  Demux/3 -> Mux8/3  "sig_z"
  Demux/1 -> Mux8/1  "sig_x"
  Demux/4 -> Mux10/1  "sig_roll"
  Mux10/1 -> [sig_ang]
  Mux8/1 -> [sig_lin]
  [sigma] -> Demux/1
  Demux/2 -> Mux8/2  "sig_y"
  [sig_lin] -> FxTESO ASGSM/10
  [sig_ang] -> FxTESO ASGSM/11
  Demux2/2 -> [pose_pitch]  "pitch"
  Demux2/3 -> [pose_yaw]  "yaw"
  Demux2/1 -> [pose_roll]  "roll"
  In Bus Element17/1 -> [Kt]
  In Bus Element16/1 -> Mux13/2
  In Bus Element15/1 -> Mux13/1
  In Bus Element14/1 -> Mux14/2
  Mux13/1 -> [error]
  Mux14/1 -> [sigma]
  Mux15/1 -> [F]
  Mux16/1 -> [qd]
  In Bus Element18/1 -> Mux16/1
  In Bus Element19/1 -> Quaternions to Rotation Angles/1  "qd"
  Quaternions to Rotation Angles/1 -> Mux16/2
  BusElementIn/1 -> [pos_hat]
  BusElementIn1/1 -> [vel_hat]
  BusElementIn2/1 -> [q_hat]
  BusElementIn3/1 -> [omega_hat]
  [pos_hat] -> Demux5/1
  In Bus Element8/1 -> [vel]
  In Bus Element9/1 -> [omega]
  ? -> Estimate/6
  [vel_hat] -> Estimate/5
  [vel] -> Estimate/4
  [omega] -> Estimate/10
  [omega_hat] -> Estimate/11
  ? -> Estimate/12
  [pos] -> Estimate/1
  [pos_hat] -> Estimate/2
  [e_hat] -> Estimate/3
  [q] -> Estimate/7  "eta"
  [q_hat] -> Estimate/8  "eta_hat"
  [q_hat_e] -> Estimate/9  "eta_hat_e"
  [q_hat] -> Quaternions to Rotation Angles3/1
  [pos] -> Demux1/1
  [pos_hat] -> Demux3/1
  Demux1/1 -> Mux17/1  "x"
  Demux3/1 -> Mux17/2  "x_hat"
  Demux1/2 -> Mux19/1  "y"
  Demux3/2 -> Mux19/2  "y_hat"
  Demux1/3 -> Mux20/1  "z"
  Demux3/3 -> Mux20/2  "z_hat"
  [BF_att] -> Demux6/1  "eta"
  Quaternions to Rotation Angles3/1 -> Demux13/1  "eta_hat"
  Mux17/1 -> real vs estimates/1
  Mux19/1 -> real vs estimates/2
  Mux20/1 -> real vs estimates/3
  Demux6/1 -> Mux21/1  "roll"
  Demux6/2 -> Mux28/1  "pitch"
  Demux6/3 -> Mux29/1  "yaw"
  Demux13/1 -> Mux21/2  "roll_hat"
  Demux13/2 -> Mux28/2  "pitch_hat"
  Demux13/3 -> Mux29/2  "yaw_hat"
  Mux21/1 -> real vs estimates/4
  Mux28/1 -> real vs estimates/5
  Mux29/1 -> real vs estimates/6
  From55/1 -> Mux33/2, Quaternions to Rotation Angles4/1
  Quaternions to Rotation Angles4/1 -> Mux33/3  "eta_hat_e"
  From53/1 -> Mux33/1
  Mux33/1 -> To Workspace6/1
  From56/1 -> To Workspace7/1
  From18/1 -> Mux2/1
  From19/1 -> Mux2/2
  From57/1 -> Mux2/3
  From58/1 -> Mux2/4
  From59/1 -> Mux2/5
  From60/1 -> Mux2/6
  Mux2/1 -> To Workspace5/1
  BusElementIn4/1 -> [e_hat]
  BusElementIn5/1 -> [q_hat_e]
  BusElementIn6/1 -> [q]

== system hexa_CAD_FxQDiff_ASGSM/6DoF_Dynamics/APC_8X3_8_Slow_Flyer_1_RIGID ==
  ReferenceFrame : sm_lib/Frames and Transforms/Reference Frame
  Solid : sm_lib/Body Elements/File Solid  ExtGeomFileName=APC 8X3.8 Slow Flyer_Valor predeterminado_sldprt.STEP  UnitType=FromFile  ExtGeomFileUnits=m  StepReaderType=HEX  ExportConvexHullGeometry=off  InertiaType=Custom  BasedOnType=DensityFromFile  Density=1000  DensityUnits=kg/m^3  Mass=smiData.Solid(8).mass  MassUnits=kg  CenterOfMass=smiData.Solid(8).CoM  CenterOfMassUnits=mm  MomentsOfInertia=smiData.Solid(8).MoI  MomentsOfInertiaUnits=kg*mm^2  ProductsOfInertia=smiData.Solid(8).PoI  ProductsOfInertiaUnits=kg*mm^2  GraphicType=FromGeometry  MarkerShape=Sphere  MarkerSize=10  GraphicVisPropType=SimpleVisualProperties  GraphicDiffuseColor=smiData.Solid(8).color  GraphicOpacity=smiData.Solid(8).opacity  GraphicSpecularColor=[0.5 0.5 0.5 1.0]  GraphicAmbientColor=[0.15 0.15 0.15 1.0]  GraphicEmissiveColor=[0.0 0.0 0.0 1.0]  GraphicShininess=75  DoExposeReferenceFrame=on  SerializedFrames=<Frames/>
  Transform : sm_lib/Frames and Transforms/Rigid Transform  RotationMethod=ArbitraryAxis  FollAlignAxisA=+X  BaseAlignAxisA=+Y  FollAlignAxisB=+Y  BaseAlignAxisB=+Z  RotationStandardAxis=+Z  RotationAngle=smiData.RigidTransform(20).angle  RotationAngleUnits=rad  RotationArbitraryAxis=smiData.RigidTransform(20).axis  RotationSequenceAxes=FollowerAxes  RotationSequence=XYX  RotationSequenceAngles=[0 0 0]  RotationSequenceAnglesUnits=deg  RotationMatrix=[1 0 0; 0 1 0; 0 0 1]  Quaternion=[1 0 0 0]  TranslationMethod=Cartesian  TranslationCartesianOffset=smiData.RigidTransform(20).translation  TranslationCartesianOffsetUnits=mm  TranslationStandardAxis=+Z  TranslationStandardOffset=0  TranslationStandardOffsetUnits=m  TranslationROffset=0  TranslationROffsetUnits=m  TranslationThetaOffset=0  TranslationThetaOffsetUnits=deg  TranslationZOffset=0  TranslationZOffsetUnits=m
  F : PMIOPort  Side=Left
  connections:
  ReferenceFrame/RConn1 -- Solid/RConn1 -- Transform/LConn1
  Transform/RConn1 -- F/RConn1

== system hexa_CAD_FxQDiff_ASGSM/6DoF_Dynamics/APC_8X3_8_Slow_Flyer_2_RIGID ==
  ReferenceFrame : sm_lib/Frames and Transforms/Reference Frame
  Solid : sm_lib/Body Elements/File Solid  ExtGeomFileName=APC 8X3.8 Slow Flyer_Valor predeterminado_sldprt.STEP  UnitType=FromFile  ExtGeomFileUnits=m  StepReaderType=HEX  ExportConvexHullGeometry=off  InertiaType=Custom  BasedOnType=DensityFromFile  Density=1000  DensityUnits=kg/m^3  Mass=smiData.Solid(8).mass  MassUnits=kg  CenterOfMass=smiData.Solid(8).CoM  CenterOfMassUnits=mm  MomentsOfInertia=smiData.Solid(8).MoI  MomentsOfInertiaUnits=kg*mm^2  ProductsOfInertia=smiData.Solid(8).PoI  ProductsOfInertiaUnits=kg*mm^2  GraphicType=FromGeometry  MarkerShape=Sphere  MarkerSize=10  GraphicVisPropType=SimpleVisualProperties  GraphicDiffuseColor=smiData.Solid(8).color  GraphicOpacity=smiData.Solid(8).opacity  GraphicSpecularColor=[0.5 0.5 0.5 1.0]  GraphicAmbientColor=[0.15 0.15 0.15 1.0]  GraphicEmissiveColor=[0.0 0.0 0.0 1.0]  GraphicShininess=75  DoExposeReferenceFrame=on  SerializedFrames=<Frames/>
  Transform : sm_lib/Frames and Transforms/Rigid Transform  RotationMethod=ArbitraryAxis  FollAlignAxisA=+X  BaseAlignAxisA=+Y  FollAlignAxisB=+Y  BaseAlignAxisB=+Z  RotationStandardAxis=+Z  RotationAngle=smiData.RigidTransform(26).angle  RotationAngleUnits=rad  RotationArbitraryAxis=smiData.RigidTransform(26).axis  RotationSequenceAxes=FollowerAxes  RotationSequence=XYX  RotationSequenceAngles=[0 0 0]  RotationSequenceAnglesUnits=deg  RotationMatrix=[1 0 0; 0 1 0; 0 0 1]  Quaternion=[1 0 0 0]  TranslationMethod=Cartesian  TranslationCartesianOffset=smiData.RigidTransform(26).translation  TranslationCartesianOffsetUnits=mm  TranslationStandardAxis=+Z  TranslationStandardOffset=0  TranslationStandardOffsetUnits=m  TranslationROffset=0  TranslationROffsetUnits=m  TranslationThetaOffset=0  TranslationThetaOffsetUnits=deg  TranslationZOffset=0  TranslationZOffsetUnits=m
  F : PMIOPort  Side=Left
  connections:
  ReferenceFrame/RConn1 -- Solid/RConn1 -- Transform/LConn1
  Transform/RConn1 -- F/RConn1

== system hexa_CAD_FxQDiff_ASGSM/6DoF_Dynamics/APC_8X3_8_Slow_Flyer_3_RIGID ==
  ReferenceFrame : sm_lib/Frames and Transforms/Reference Frame
  Solid : sm_lib/Body Elements/File Solid  ExtGeomFileName=APC 8X3.8 Slow Flyer_Valor predeterminado_sldprt.STEP  UnitType=FromFile  ExtGeomFileUnits=m  StepReaderType=HEX  ExportConvexHullGeometry=off  InertiaType=Custom  BasedOnType=DensityFromFile  Density=1000  DensityUnits=kg/m^3  Mass=smiData.Solid(8).mass  MassUnits=kg  CenterOfMass=smiData.Solid(8).CoM  CenterOfMassUnits=mm  MomentsOfInertia=smiData.Solid(8).MoI  MomentsOfInertiaUnits=kg*mm^2  ProductsOfInertia=smiData.Solid(8).PoI  ProductsOfInertiaUnits=kg*mm^2  GraphicType=FromGeometry  MarkerShape=Sphere  MarkerSize=10  GraphicVisPropType=SimpleVisualProperties  GraphicDiffuseColor=smiData.Solid(8).color  GraphicOpacity=smiData.Solid(8).opacity  GraphicSpecularColor=[0.5 0.5 0.5 1.0]  GraphicAmbientColor=[0.15 0.15 0.15 1.0]  GraphicEmissiveColor=[0.0 0.0 0.0 1.0]  GraphicShininess=75  DoExposeReferenceFrame=on  SerializedFrames=<Frames/>
  Transform : sm_lib/Frames and Transforms/Rigid Transform  RotationMethod=ArbitraryAxis  FollAlignAxisA=+X  BaseAlignAxisA=+Y  FollAlignAxisB=+Y  BaseAlignAxisB=+Z  RotationStandardAxis=+Z  RotationAngle=smiData.RigidTransform(28).angle  RotationAngleUnits=rad  RotationArbitraryAxis=smiData.RigidTransform(28).axis  RotationSequenceAxes=FollowerAxes  RotationSequence=XYX  RotationSequenceAngles=[0 0 0]  RotationSequenceAnglesUnits=deg  RotationMatrix=[1 0 0; 0 1 0; 0 0 1]  Quaternion=[1 0 0 0]  TranslationMethod=Cartesian  TranslationCartesianOffset=smiData.RigidTransform(28).translation  TranslationCartesianOffsetUnits=mm  TranslationStandardAxis=+Z  TranslationStandardOffset=0  TranslationStandardOffsetUnits=m  TranslationROffset=0  TranslationROffsetUnits=m  TranslationThetaOffset=0  TranslationThetaOffsetUnits=deg  TranslationZOffset=0  TranslationZOffsetUnits=m
  F : PMIOPort  Side=Left
  connections:
  ReferenceFrame/RConn1 -- Solid/RConn1 -- Transform/LConn1
  Transform/RConn1 -- F/RConn1

== system hexa_CAD_FxQDiff_ASGSM/6DoF_Dynamics/APC_8X3_8_Slow_Flyer_4_RIGID ==
  ReferenceFrame : sm_lib/Frames and Transforms/Reference Frame
  Solid : sm_lib/Body Elements/File Solid  ExtGeomFileName=APC 8X3.8 Slow Flyer_Valor predeterminado_sldprt.STEP  UnitType=FromFile  ExtGeomFileUnits=m  StepReaderType=HEX  ExportConvexHullGeometry=off  InertiaType=Custom  BasedOnType=DensityFromFile  Density=1000  DensityUnits=kg/m^3  Mass=smiData.Solid(8).mass  MassUnits=kg  CenterOfMass=smiData.Solid(8).CoM  CenterOfMassUnits=mm  MomentsOfInertia=smiData.Solid(8).MoI  MomentsOfInertiaUnits=kg*mm^2  ProductsOfInertia=smiData.Solid(8).PoI  ProductsOfInertiaUnits=kg*mm^2  GraphicType=FromGeometry  MarkerShape=Sphere  MarkerSize=10  GraphicVisPropType=SimpleVisualProperties  GraphicDiffuseColor=smiData.Solid(8).color  GraphicOpacity=smiData.Solid(8).opacity  GraphicSpecularColor=[0.5 0.5 0.5 1.0]  GraphicAmbientColor=[0.15 0.15 0.15 1.0]  GraphicEmissiveColor=[0.0 0.0 0.0 1.0]  GraphicShininess=75  DoExposeReferenceFrame=on  SerializedFrames=<Frames/>
  Transform : sm_lib/Frames and Transforms/Rigid Transform  RotationMethod=ArbitraryAxis  FollAlignAxisA=+X  BaseAlignAxisA=+Y  FollAlignAxisB=+Y  BaseAlignAxisB=+Z  RotationStandardAxis=+Z  RotationAngle=smiData.RigidTransform(34).angle  RotationAngleUnits=rad  RotationArbitraryAxis=smiData.RigidTransform(34).axis  RotationSequenceAxes=FollowerAxes  RotationSequence=XYX  RotationSequenceAngles=[0 0 0]  RotationSequenceAnglesUnits=deg  RotationMatrix=[1 0 0; 0 1 0; 0 0 1]  Quaternion=[1 0 0 0]  TranslationMethod=Cartesian  TranslationCartesianOffset=smiData.RigidTransform(34).translation  TranslationCartesianOffsetUnits=mm  TranslationStandardAxis=+Z  TranslationStandardOffset=0  TranslationStandardOffsetUnits=m  TranslationROffset=0  TranslationROffsetUnits=m  TranslationThetaOffset=0  TranslationThetaOffsetUnits=deg  TranslationZOffset=0  TranslationZOffsetUnits=m
  F : PMIOPort  Side=Left
  connections:
  ReferenceFrame/RConn1 -- Solid/RConn1 -- Transform/LConn1
  Transform/RConn1 -- F/RConn1

== system hexa_CAD_FxQDiff_ASGSM/6DoF_Dynamics/APC_8X3_8_Slow_Flyer_5_RIGID ==
  ReferenceFrame : sm_lib/Frames and Transforms/Reference Frame
  Solid : sm_lib/Body Elements/File Solid  ExtGeomFileName=APC 8X3.8 Slow Flyer_Valor predeterminado_sldprt.STEP  UnitType=FromFile  ExtGeomFileUnits=m  StepReaderType=HEX  ExportConvexHullGeometry=off  InertiaType=Custom  BasedOnType=DensityFromFile  Density=1000  DensityUnits=kg/m^3  Mass=smiData.Solid(8).mass  MassUnits=kg  CenterOfMass=smiData.Solid(8).CoM  CenterOfMassUnits=mm  MomentsOfInertia=smiData.Solid(8).MoI  MomentsOfInertiaUnits=kg*mm^2  ProductsOfInertia=smiData.Solid(8).PoI  ProductsOfInertiaUnits=kg*mm^2  GraphicType=FromGeometry  MarkerShape=Sphere  MarkerSize=10  GraphicVisPropType=SimpleVisualProperties  GraphicDiffuseColor=smiData.Solid(8).color  GraphicOpacity=smiData.Solid(8).opacity  GraphicSpecularColor=[0.5 0.5 0.5 1.0]  GraphicAmbientColor=[0.15 0.15 0.15 1.0]  GraphicEmissiveColor=[0.0 0.0 0.0 1.0]  GraphicShininess=75  DoExposeReferenceFrame=on  SerializedFrames=<Frames/>
  Transform : sm_lib/Frames and Transforms/Rigid Transform  RotationMethod=ArbitraryAxis  FollAlignAxisA=+X  BaseAlignAxisA=+Y  FollAlignAxisB=+Y  BaseAlignAxisB=+Z  RotationStandardAxis=+Z  RotationAngle=smiData.RigidTransform(36).angle  RotationAngleUnits=rad  RotationArbitraryAxis=smiData.RigidTransform(36).axis  RotationSequenceAxes=FollowerAxes  RotationSequence=XYX  RotationSequenceAngles=[0 0 0]  RotationSequenceAnglesUnits=deg  RotationMatrix=[1 0 0; 0 1 0; 0 0 1]  Quaternion=[1 0 0 0]  TranslationMethod=Cartesian  TranslationCartesianOffset=smiData.RigidTransform(36).translation  TranslationCartesianOffsetUnits=mm  TranslationStandardAxis=+Z  TranslationStandardOffset=0  TranslationStandardOffsetUnits=m  TranslationROffset=0  TranslationROffsetUnits=m  TranslationThetaOffset=0  TranslationThetaOffsetUnits=deg  TranslationZOffset=0  TranslationZOffsetUnits=m
  F : PMIOPort  Side=Left
  connections:
  ReferenceFrame/RConn1 -- Solid/RConn1 -- Transform/LConn1
  Transform/RConn1 -- F/RConn1

== system hexa_CAD_FxQDiff_ASGSM/6DoF_Dynamics/APC_8X3_8_Slow_Flyer_6_RIGID ==
  ReferenceFrame : sm_lib/Frames and Transforms/Reference Frame
  Solid : sm_lib/Body Elements/File Solid  ExtGeomFileName=APC 8X3.8 Slow Flyer_Valor predeterminado_sldprt.STEP  UnitType=FromFile  ExtGeomFileUnits=m  StepReaderType=HEX  ExportConvexHullGeometry=off  InertiaType=Custom  BasedOnType=DensityFromFile  Density=1000  DensityUnits=kg/m^3  Mass=smiData.Solid(8).mass  MassUnits=kg  CenterOfMass=smiData.Solid(8).CoM  CenterOfMassUnits=mm  MomentsOfInertia=smiData.Solid(8).MoI  MomentsOfInertiaUnits=kg*mm^2  ProductsOfInertia=smiData.Solid(8).PoI  ProductsOfInertiaUnits=kg*mm^2  GraphicType=FromGeometry  MarkerShape=Sphere  MarkerSize=10  GraphicVisPropType=SimpleVisualProperties  GraphicDiffuseColor=smiData.Solid(8).color  GraphicOpacity=smiData.Solid(8).opacity  GraphicSpecularColor=[0.5 0.5 0.5 1.0]  GraphicAmbientColor=[0.15 0.15 0.15 1.0]  GraphicEmissiveColor=[0.0 0.0 0.0 1.0]  GraphicShininess=75  DoExposeReferenceFrame=on  SerializedFrames=<Frames/>
  Transform : sm_lib/Frames and Transforms/Rigid Transform  RotationMethod=ArbitraryAxis  FollAlignAxisA=+X  BaseAlignAxisA=+Y  FollAlignAxisB=+Y  BaseAlignAxisB=+Z  RotationStandardAxis=+Z  RotationAngle=smiData.RigidTransform(42).angle  RotationAngleUnits=rad  RotationArbitraryAxis=smiData.RigidTransform(42).axis  RotationSequenceAxes=FollowerAxes  RotationSequence=XYX  RotationSequenceAngles=[0 0 0]  RotationSequenceAnglesUnits=deg  RotationMatrix=[1 0 0; 0 1 0; 0 0 1]  Quaternion=[1 0 0 0]  TranslationMethod=Cartesian  TranslationCartesianOffset=smiData.RigidTransform(42).translation  TranslationCartesianOffsetUnits=mm  TranslationStandardAxis=+Z  TranslationStandardOffset=0  TranslationStandardOffsetUnits=m  TranslationROffset=0  TranslationROffsetUnits=m  TranslationThetaOffset=0  TranslationThetaOffsetUnits=deg  TranslationZOffset=0  TranslationZOffsetUnits=m
  F : PMIOPort  Side=Left
  connections:
  ReferenceFrame/RConn1 -- Solid/RConn1 -- Transform/LConn1
  Transform/RConn1 -- F/RConn1
